simulink model "SRM_ZETA_PID"  (R2020a)
settings: Solver=VariableStepAuto  StartTime=0.0  StopTime=10.0  RelTol=1e-3
undefined symbols (not defined in the file): DiscIntNeverNeededParam, find_system, K, TL, Ts
libraries: powerlib x59
settings Model: Creator=mahfo  LastModifiedBy=mahfo

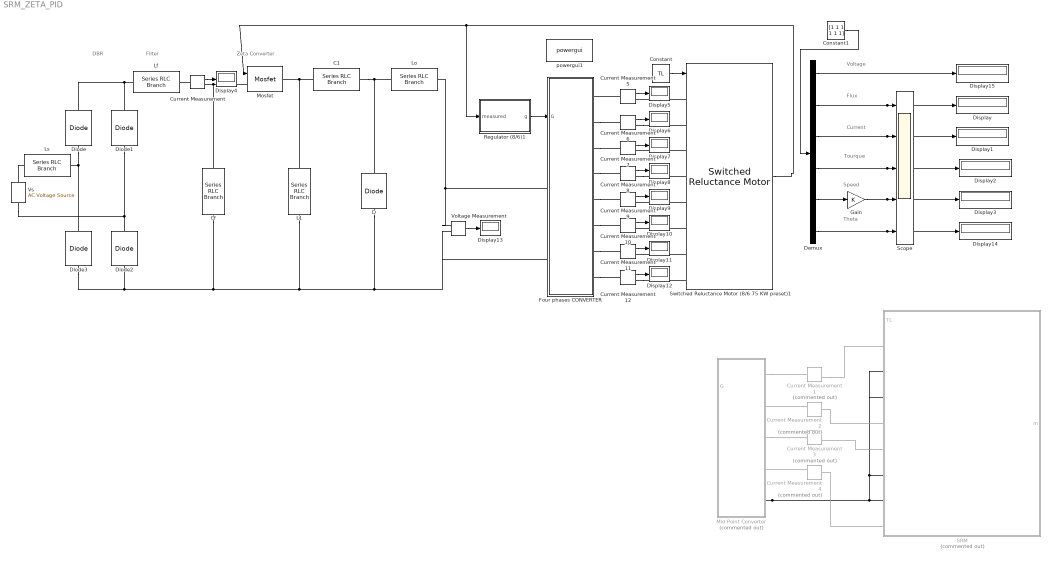
== system SRM_ZETA_PID ==
  note: Flux
  note: DBR
  note: Filter
  note: Zeta Converter
  note: Speed
  note: Theta
  note: Current
  note: Tourque
  note: Voltage
  C1 : powerlib/Elements/Series RLC Branch  LConnTagsString=__new0  RConnTagsString=__new0  BranchType=C  Resistance=1  Inductance=1e-3  SetiL0=off  InitialCurrent=0  Capacitance=1e-6  Setx0=off  InitialVoltage=0  Measurements=None
  Cf : powerlib/Elements/Series RLC Branch  LConnTagsString=__new0  RConnTagsString=__new0  BranchType=C  Resistance=1  Inductance=1e-3  SetiL0=off  InitialCurrent=0  Capacitance=1e-6  Setx0=off  InitialVoltage=0  Measurements=None
  Constant : Constant  Value=TL
  Constant1 : Constant  Value=[1 1 1 1 1 1]
  Current Measurement{,5..12} (9 alike) : powerlib/Measurements/Current Measurement  PhasorSimulation=off  OutputType=Complex  PSBequivalent=0
  Current Measurement{1..4} (4 alike) : powerlib/Measurements/Current Measurement  Commented=on  PhasorSimulation=off  OutputType=Complex  PSBequivalent=0
  D : powerlib/Power Electronics/Diode  Ron=0.001  Lon=0  Vf=0.8  IC=0  UseSnubber=0  Rs=500  Cs=250e-9  Measurements=off
  Demux : Demux  Outputs=6
  Diode{,1..3} (4 alike) : powerlib/Power Electronics/Diode  Ron=0.001  Lon=0  Vf=0.8  IC=0  UseSnubber=0  Rs=500  Cs=250e-9  Measurements=off
  Display{,1..15} (16 alike) : Display
  Four phases CONVERTER : Subsystem  LoadFcn=find_system(gcs,'FollowLinks', 'on', 'LookUnderMasks', 'all');
  Gain : Gain  Gain=K
  L1 : powerlib/Elements/Series RLC Branch  LConnTagsString=__new0  RConnTagsString=__new0  BranchType=L  Resistance=1  Inductance=1e-3  SetiL0=off  InitialCurrent=0  Capacitance=1e-6  Setx0=off  InitialVoltage=0  Measurements=None
  Lf : powerlib/Elements/Series RLC Branch  LConnTagsString=__new0  RConnTagsString=__new0  BranchType=L  Resistance=1  Inductance=1e-3  SetiL0=off  InitialCurrent=0  Capacitance=1e-6  Setx0=off  InitialVoltage=0  Measurements=None
  Lo : powerlib/Elements/Series RLC Branch  LConnTagsString=__new0  RConnTagsString=__new0  BranchType=L  Resistance=1  Inductance=1e-3  SetiL0=off  InitialCurrent=0  Capacitance=1e-6  Setx0=off  InitialVoltage=0  Measurements=None
  Ls : powerlib/Elements/Series RLC Branch  LConnTagsString=__new0  RConnTagsString=__new0  BranchType=L  Resistance=1  Inductance=1e-3  SetiL0=off  InitialCurrent=0  Capacitance=1e-6  Setx0=off  InitialVoltage=0  Measurements=None
  Mid Point Converter : Subsystem  Commented=on
  Mosfet : powerlib/Power Electronics/Mosfet  Ron=0.1  Lon=0  Rd=0.01  Vfd=0  IC=0  Rs=1e5  Cs=inf  Measurements=off
  Regulator (8/6)1 : Subsystem  mask{Iref=50, initpos=[0,-15,-30,-45], TurnOn=37.5, TurnOff=52.5}
      mask prompts: Iref "Reference current"; initpos "initial positions"; TurnOn "Turn-on angle (deg)"; TurnOff "Turn-off angle (deg)"
  SRM : Subsystem  Commented=on
      mask Display: image('F:\Semester 10\Electric Drives\Project\SRM.png'); % Use "Edit Image" on toolstrip to change.
  Scope : Scope  NumInputPorts=5
  Switched Reluctance Motor (8/6 75 KW preset)1 : powerlib/Machines/Switched Reluctance Motor  MachineType="8/6  (75 kw preset model)"  StatorResistance=0.05  Inertia=0.01  Friction=0.005  InitialSpeed=[0,0]  TsPowergui=0  TsBlock=Ts  MachineModel=Specific model  Lq=0.67e-3  Ld=23.6e-3  Lsat=0.15e-3  MaximumCurrent=450  MaximumFluxLinkage=0.486  Source=Dialog  MagnetisationCharacteristic=FTBL  RotorAngleVector=RotorAngles  StatorCurrentVector=StatorCurrents  PlotCurves=off
      settings: SourceProductBaseCode=MT,PS
  Voltage Measurement : powerlib/Measurements/Voltage Measurement  PhasorSimulation=off  OutputType=Complex  PSBequivalent=0
  Vs : powerlib/Electrical Sources/AC Voltage Source  Amplitude=240  Phase=0  Frequency=60  SampleTime=0  Measurements=None  BusType=swing  Pref=10e3  Qref=0  Qmin=-inf  Qmax=+inf
  powergui1 : powerlib/powergui  Priority=1  SimulationMode=Discrete  SampleTime=50e-6  frequency=60  Iterations=50  frequencyindice=60  Pbase=100e6  ErrMax=1e-4  UnitsV=kV  UnitsW=MW  buscounter=0  FunctionMessages=off  echomessages=off  EnableUseOfTLC=off  CurrentSourceSwitches=off  DisableSnubberDevices=off  DisableRonSwitches=off  DisableVfSwitches=off  DisplayEquations=off  AutomaticDiscreteSolvers=off  SolverType=Tustin/Backward Euler (TBE)  Interpol=off  ExternalGateDelay=off  methode=off  Ts=100  x0status=blocks  SPID=on  SwTol=0  HookPort=off  NonlinearTolerance=1e-4  nMaxIteration=100  ContinueOnMaxIteration=off  RestoreLinks=warning  ResistiveCurrentMeasurement=off  Frange=[0:2:500]  Ylog=off  Xlog=on  ShowGrid=off  save=off  variable=ZData  structure=0  ZoomFFT=off  StartTime=0.0  cycles=1  DisplayStyle=1  fundamental=60  FreqAxis=off  MaxFrequency=1000  frequencyindicesteady=1  RmsSteady=1  display=off
  wires:
  Switched Reluctance Motor (8/6 75 KW preset)1/1 -> Regulator (8/6)1/1(measured), Mosfet/1
  Gain/1 -> Display3/1, Scope/4
  Regulator (8/6)1/1(g) -> Four phases CONVERTER/1(G)
  Constant/1 -> Switched Reluctance Motor (8/6 75 KW preset)1/1
  Current Measurement/1 -> Display4/1
  Current Measurement5/1 -> Display5/1
  Current Measurement6/1 -> Display6/1
  Current Measurement7/1 -> Display7/1
  Current Measurement8/1 -> Display8/1
  Current Measurement9/1 -> Display9/1
  Current Measurement10/1 -> Display10/1
  Current Measurement11/1 -> Display11/1
  Current Measurement12/1 -> Display12/1
  Voltage Measurement/1 -> Display13/1
  Demux/6 -> Display14/1, Scope/5
  Demux/5 -> Gain/1
  Demux/4 -> Display2/1, Scope/3
  Demux/3 -> Display1/1, Scope/2
  Demux/2 -> Display/1, Scope/1
  Demux/1 -> Display15/1
  Constant1/1 -> Demux/1
  connections:
  Vs/RConn1 -- Ls/LConn1
  Diode/LConn1 -- Ls/RConn1 -- Diode3/RConn1
  Diode1/LConn1 -- Vs/LConn1 -- Diode2/RConn1
  Diode/RConn1 -- Diode1/RConn1 -- Lf/LConn1
  Diode3/LConn1 -- Cf/RConn1 -- Voltage Measurement/LConn2 -- Four phases CONVERTER/LConn2 -- D/LConn1 -- L1/LConn1 -- Diode2/LConn1
  Current Measurement/LConn1 -- Lf/RConn1
  Current Measurement/RConn1 -- Cf/LConn1 -- Mosfet/LConn1
  L1/RConn1 -- C1/LConn1 -- Mosfet/RConn1
  Lo/LConn1 -- C1/RConn1 -- D/RConn1
  Voltage Measurement/LConn1 -- Lo/RConn1 -- Four phases CONVERTER/LConn1
  Mid Point Converter/RConn5 -- SRM/LConn7 -- SRM/LConn6 -- SRM/LConn3 -- SRM/LConn2
  Current Measurement1/RConn1 -- SRM/LConn1
  Current Measurement2/RConn1 -- Mid Point Converter/RConn2
  SRM/LConn4 -- Current Measurement2/LConn1
  SRM/LConn8 -- Current Measurement4/LConn1
  SRM/LConn5 -- Current Measurement3/RConn1
  Current Measurement4/RConn1 -- Mid Point Converter/RConn4
  Mid Point Converter/RConn3 -- Current Measurement3/LConn1
  Mid Point Converter/RConn1 -- Current Measurement1/LConn1
  Current Measurement5/LConn1 -- Four phases CONVERTER/RConn1
  Switched Reluctance Motor (8/6 75 KW preset)1/LConn1 -- Current Measurement5/RConn1
  Four phases CONVERTER/RConn2 -- Current Measurement6/LConn1
  Current Measurement6/RConn1 -- Switched Reluctance Motor (8/6 75 KW preset)1/LConn2
  Four phases CONVERTER/RConn4 -- Current Measurement8/LConn1
  Switched Reluctance Motor (8/6 75 KW preset)1/LConn3 -- Current Measurement7/RConn1
  Current Measurement8/RConn1 -- Switched Reluctance Motor (8/6 75 KW preset)1/LConn4
  Four phases CONVERTER/RConn3 -- Current Measurement7/LConn1
  Current Measurement12/RConn1 -- Switched Reluctance Motor (8/6 75 KW preset)1/LConn8
  Switched Reluctance Motor (8/6 75 KW preset)1/LConn7 -- Current Measurement11/RConn1
  Four phases CONVERTER/RConn8 -- Current Measurement12/LConn1
  Four phases CONVERTER/RConn6 -- Current Measurement10/LConn1
  Four phases CONVERTER/RConn7 -- Current Measurement11/LConn1
  Switched Reluctance Motor (8/6 75 KW preset)1/LConn5 -- Current Measurement9/RConn1
  Switched Reluctance Motor (8/6 75 KW preset)1/LConn6 -- Current Measurement10/RConn1
  Four phases CONVERTER/RConn5 -- Current Measurement9/LConn1

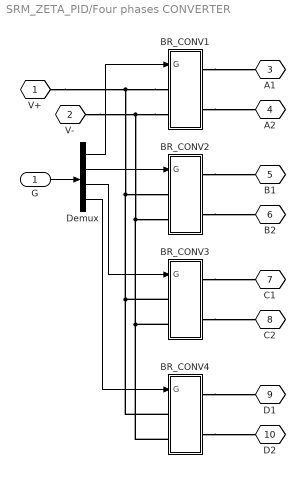
== system SRM_ZETA_PID/Four phases CONVERTER ==
  G : Inport
  BR_CONV1 : Subsystem
  BR_CONV2 : Subsystem
  BR_CONV3 : Subsystem
  BR_CONV4 : Subsystem
  Demux : Demux
      settings: DisplayOption=none
  V+ : PMIOPort  Tag=PMCPort  Side=Left
  V- : PMIOPort  Tag=PMCPort  Port=2  Side=Left
  A1 : PMIOPort  Tag=PMCPort  Port=3  Side=Right
  A2 : PMIOPort  Tag=PMCPort  Port=4  Side=Right
  B1 : PMIOPort  Tag=PMCPort  Port=5  Side=Right
  B2 : PMIOPort  Tag=PMCPort  Port=6  Side=Right
  C1 : PMIOPort  Tag=PMCPort  Port=7  Side=Right
  C2 : PMIOPort  Tag=PMCPort  Port=8  Side=Right
  D1 : PMIOPort  Tag=PMCPort  Port=9  Side=Right
  D2 : PMIOPort  Tag=PMCPort  Port=10  Side=Right
  wires:
  Demux/4 -> BR_CONV4/1(G)
  Demux/3 -> BR_CONV3/1(G)
  Demux/1 -> BR_CONV1/1(G)
  Demux/2 -> BR_CONV2/1(G)
  G/1 -> Demux/1
  connections:
  BR_CONV4/RConn1 -- D1/RConn1
  BR_CONV4/RConn2 -- D2/RConn1
  BR_CONV3/RConn2 -- C2/RConn1
  BR_CONV3/RConn1 -- C1/RConn1
  BR_CONV2/RConn2 -- B2/RConn1
  BR_CONV2/RConn1 -- B1/RConn1
  BR_CONV1/RConn2 -- A2/RConn1
  BR_CONV1/RConn1 -- A1/RConn1
  BR_CONV1/LConn2 -- V-/RConn1 -- BR_CONV3/LConn2 -- BR_CONV4/LConn2 -- BR_CONV2/LConn2
  BR_CONV1/LConn1 -- V+/RConn1 -- BR_CONV3/LConn1 -- BR_CONV4/LConn1 -- BR_CONV2/LConn1

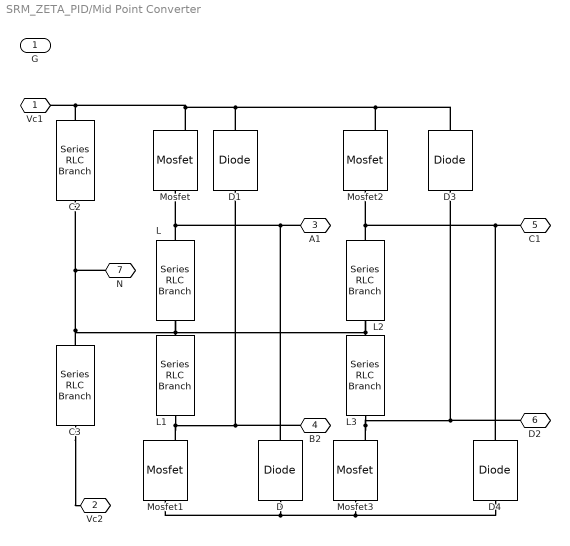
== system SRM_ZETA_PID/Mid Point Converter ==
  G : Inport
  C2 : powerlib/Elements/Series RLC Branch  LConnTagsString=__new0  RConnTagsString=__new0  BranchType=C  Resistance=1  Inductance=1e-3  SetiL0=off  InitialCurrent=0  Capacitance=1e-6  Setx0=off  InitialVoltage=0  Measurements=None
  C3 : powerlib/Elements/Series RLC Branch  LConnTagsString=__new0  RConnTagsString=__new0  BranchType=C  Resistance=1  Inductance=1e-3  SetiL0=off  InitialCurrent=0  Capacitance=1e-6  Setx0=off  InitialVoltage=0  Measurements=None
  D{,1,3..4} (4 alike) : powerlib/Power Electronics/Diode  Ron=0.001  Lon=0  Vf=0.8  IC=0  UseSnubber=0  Rs=500  Cs=250e-9  Measurements=off
  L{,1..3} (4 alike) : powerlib/Elements/Series RLC Branch  LConnTagsString=__new0  RConnTagsString=__new0  BranchType=L  Resistance=1  Inductance=1e-3  SetiL0=off  InitialCurrent=0  Capacitance=1e-6  Setx0=off  InitialVoltage=0  Measurements=None
  Mosfet{,1..3} (4 alike) : powerlib/Power Electronics/Mosfet  Ron=0.1  Lon=0  Rd=0.01  Vfd=0  IC=0  Rs=1e5  Cs=inf  Measurements=off
  Vc1 : PMIOPort  Side=Left
  Vc2 : PMIOPort  Port=2  Side=Left
  A1 : PMIOPort  Port=3  Side=Right
  B2 : PMIOPort  Port=4  Side=Right
  C1 : PMIOPort  Port=5  Side=Right
  D2 : PMIOPort  Port=6  Side=Right
  N : PMIOPort  Port=7  Side=Right
  connections:
  D1/RConn1 -- Vc1/RConn1 -- C2/LConn1 -- Mosfet/LConn1 -- Mosfet2/LConn1 -- D3/RConn1
  C3/RConn1 -- Vc2/RConn1
  A1/RConn1 -- D/RConn1 -- L/LConn1 -- Mosfet/RConn1
  D1/LConn1 -- L1/LConn1 -- Mosfet1/LConn1 -- B2/RConn1
  D4/RConn1 -- C1/RConn1 -- L2/LConn1 -- Mosfet2/RConn1
  D/LConn1 -- Mosfet1/RConn1 -- Mosfet3/RConn1 -- D4/LConn1
  D3/LConn1 -- L3/LConn1 -- Mosfet3/LConn1 -- D2/RConn1
  N/RConn1 -- C2/RConn1 -- C3/LConn1 -- L1/RConn1 -- L3/RConn1 -- L2/RConn1

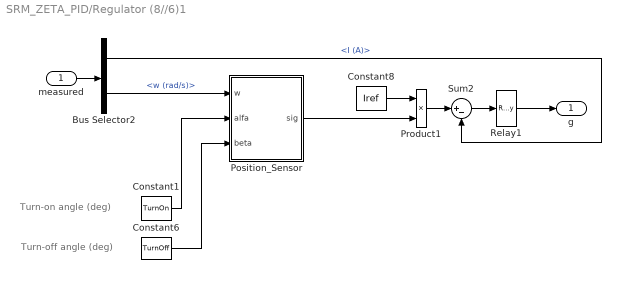
== system SRM_ZETA_PID/Regulator (8//6)1 ==
  note: Turn-on angle (deg)
  note: Turn-off angle (deg)
  measured : Inport
  Bus Selector2 : BusSelector  OutputSignals=I (A),w (rad/s)
  Constant1 : Constant  Value=TurnOn
  Constant6 : Constant  Value=TurnOff
  Constant8 : Constant  Value=Iref
  Position_Sensor : Subsystem
  Product1 : Product  SaturateOnIntegerOverflow=on  OutDataTypeStr=Inherit: Same as first input
  Relay1 : Relay  OnSwitchValue=5  OffSwitchValue=-5  SampleTime=Ts
  Sum2 : Sum  Inputs=|+-  SaturateOnIntegerOverflow=on
  g : Outport  VectorParamsAs1DForOutWhenUnconnected=off
  wires:
  Bus Selector2/2 -> Position_Sensor/1(w)  "<w (rad/s)>"
  Bus Selector2/1 -> Sum2/2  "<I (A)>"
  measured/1 -> Bus Selector2/1
  Relay1/1 -> g/1
  Position_Sensor/1(sig) -> Product1/2
  Constant8/1 -> Product1/1
  Product1/1 -> Sum2/1
  Sum2/1 -> Relay1/1
  Constant6/1 -> Position_Sensor/3(beta)
  Constant1/1 -> Position_Sensor/2(alfa)

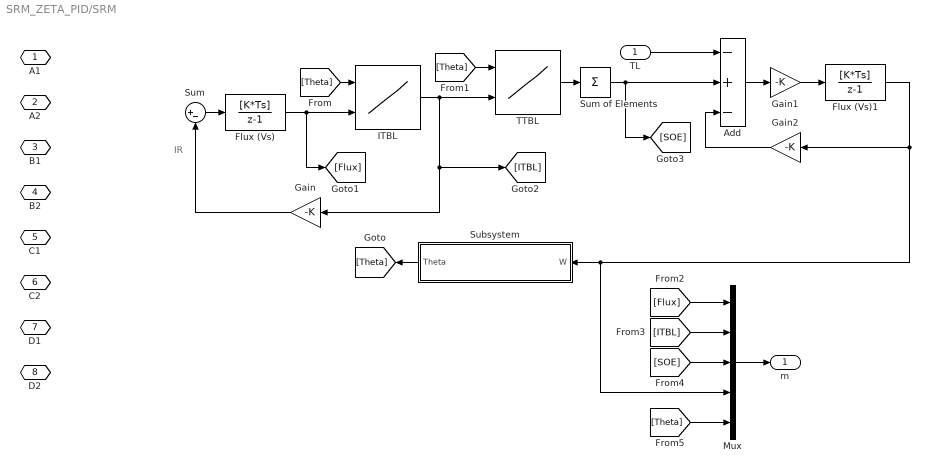
== system SRM_ZETA_PID/SRM ==
  note: IR
  TL : Inport
  Add : Sum  Inputs=-+-
  Flux (Vs) : DiscreteTransferFcn  Numerator=[K*Ts]  Denominator=[1 -1]
  Flux (Vs)1 : DiscreteTransferFcn  Numerator=[K*Ts]  Denominator=[1 -1]
  Gain : Gain  Gain=-K
  Gain1 : Gain  Gain=-K
  Gain2 : Gain  Gain=-K
  ITBL : Lookup_n-D  BreakpointsForDimension1=[1:3]  BreakpointsForDimension2=[1:3]  InternalRulePriority=Speed  RndMeth=Simplest  InputSameDT=on
  Mux : Mux  Inputs=5
  Subsystem : Subsystem
  Sum : Sum  Inputs=|+-
  Sum of Elements : Sum  Inputs=+
  TTBL : Lookup_n-D  BreakpointsForDimension1=[1:3]  BreakpointsForDimension2=[1:3]  InternalRulePriority=Speed  RndMeth=Simplest  InputSameDT=on
  A1 : PMIOPort  Side=Left
  A2 : PMIOPort  Port=2  Side=Left
  B1 : PMIOPort  Port=3  Side=Left
  B2 : PMIOPort  Port=4  Side=Left
  C1 : PMIOPort  Port=5  Side=Left
  C2 : PMIOPort  Port=6  Side=Left
  D1 : PMIOPort  Port=7  Side=Left
  D2 : PMIOPort  Port=8  Side=Left
  m : Outport
  wires:
  Sum/1 -> Flux (Vs)/1
  Flux (Vs)/1 -> [Flux], ITBL/2
  ITBL/1 -> Gain/1, [ITBL], TTBL/2
  TTBL/1 -> Sum of Elements/1
  Gain/1 -> Sum/2
  Sum of Elements/1 -> [SOE], Add/2
  TL/1 -> Add/1
  Add/1 -> Gain1/1
  Gain1/1 -> Flux (Vs)1/1
  Flux (Vs)1/1 -> Mux/4, Subsystem/1(W), Gain2/1
  Gain2/1 -> Add/3
  [Theta] -> ITBL/1
  Subsystem/1(Theta) -> [Theta]
  [Theta] -> TTBL/1
  [Flux] -> Mux/1
  [ITBL] -> Mux/2
  [SOE] -> Mux/3
  [Theta] -> Mux/5
  Mux/1 -> m/1

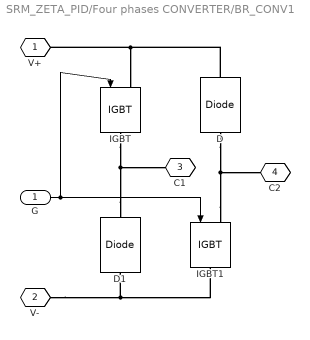
== system SRM_ZETA_PID/Four phases CONVERTER/BR_CONV1 ==
  G : Inport
  D : powerlib/Power Electronics/Diode  Ron=1e-3  Lon=0  Vf=0.8  IC=0  UseSnubber=off  Rs=1000  Cs=inf  Measurements=off
      settings: SourceProductBaseCode=MT,PS
  D1 : powerlib/Power Electronics/Diode  Ron=1e-3  Lon=0  Vf=0.8  IC=0  UseSnubber=off  Rs=1000  Cs=inf  Measurements=off
      settings: SourceProductBaseCode=MT,PS
  IGBT : powerlib/Power Electronics/IGBT  Ron=1e-3  Lon=0  Vf=1  Tf=0  Tt=0  IC=0  Rs=200  Cs=0.1e-6  Measurements=off
      settings: SourceProductBaseCode=MT,PS
  IGBT1 : powerlib/Power Electronics/IGBT  Ron=1e-3  Lon=0  Vf=1  Tf=0  Tt=0  IC=0  Rs=200  Cs=0.1e-6  Measurements=off
      settings: SourceProductBaseCode=MT,PS
  V+ : PMIOPort  Tag=PMCPort  Side=Left
  V- : PMIOPort  Tag=PMCPort  Port=2  Side=Left
  C1 : PMIOPort  Tag=PMCPort  Port=3  Side=Right
  C2 : PMIOPort  Tag=PMCPort  Port=4  Side=Right
  wires:
  G/1 -> IGBT/1, IGBT1/1
  connections:
  D1/LConn1 -- V-/RConn1 -- IGBT1/RConn1
  IGBT1/LConn1 -- D/LConn1 -- C2/RConn1
  D1/RConn1 -- IGBT/RConn1 -- C1/RConn1
  D/RConn1 -- V+/RConn1 -- IGBT/LConn1

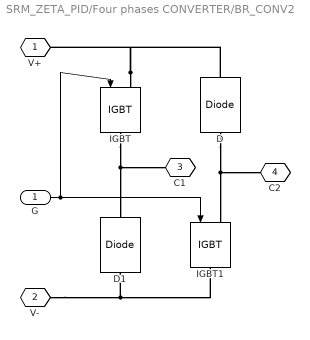
== system SRM_ZETA_PID/Four phases CONVERTER/BR_CONV2 ==
  G : Inport
  D : powerlib/Power Electronics/Diode  Ron=1e-3  Lon=0  Vf=0.8  IC=0  UseSnubber=off  Rs=1000  Cs=inf  Measurements=off
      settings: SourceProductBaseCode=MT,PS
  D1 : powerlib/Power Electronics/Diode  Ron=1e-3  Lon=0  Vf=0.8  IC=0  UseSnubber=off  Rs=1000  Cs=inf  Measurements=off
      settings: SourceProductBaseCode=MT,PS
  IGBT : powerlib/Power Electronics/IGBT  Ron=1e-3  Lon=0  Vf=1  Tf=0  Tt=0  IC=0  Rs=200  Cs=0.1e-6  Measurements=off
      settings: SourceProductBaseCode=MT,PS
  IGBT1 : powerlib/Power Electronics/IGBT  Ron=1e-3  Lon=0  Vf=1  Tf=0  Tt=0  IC=0  Rs=200  Cs=0.1e-6  Measurements=off
      settings: SourceProductBaseCode=MT,PS
  V+ : PMIOPort  Tag=PMCPort  Side=Left
  V- : PMIOPort  Tag=PMCPort  Port=2  Side=Left
  C1 : PMIOPort  Tag=PMCPort  Port=3  Side=Right
  C2 : PMIOPort  Tag=PMCPort  Port=4  Side=Right
  wires:
  G/1 -> IGBT1/1, IGBT/1
  connections:
  IGBT/LConn1 -- V+/RConn1 -- D/RConn1
  IGBT/RConn1 -- D1/RConn1 -- C1/RConn1
  D/LConn1 -- IGBT1/LConn1 -- C2/RConn1
  V-/RConn1 -- D1/LConn1 -- IGBT1/RConn1

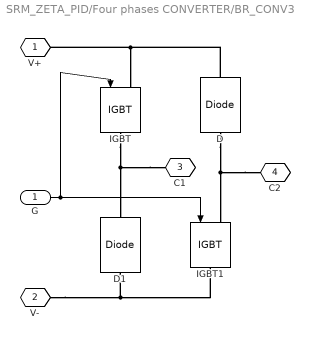
== system SRM_ZETA_PID/Four phases CONVERTER/BR_CONV3 ==
  G : Inport
  D : powerlib/Power Electronics/Diode  Ron=1e-3  Lon=0  Vf=0.8  IC=0  UseSnubber=off  Rs=1000  Cs=inf  Measurements=off
      settings: SourceProductBaseCode=MT,PS
  D1 : powerlib/Power Electronics/Diode  Ron=1e-3  Lon=0  Vf=0.8  IC=0  UseSnubber=off  Rs=1000  Cs=inf  Measurements=off
      settings: SourceProductBaseCode=MT,PS
  IGBT : powerlib/Power Electronics/IGBT  Ron=1e-3  Lon=0  Vf=1  Tf=0  Tt=0  IC=0  Rs=200  Cs=0.1e-6  Measurements=off
      settings: SourceProductBaseCode=MT,PS
  IGBT1 : powerlib/Power Electronics/IGBT  Ron=1e-3  Lon=0  Vf=1  Tf=0  Tt=0  IC=0  Rs=200  Cs=0.1e-6  Measurements=off
      settings: SourceProductBaseCode=MT,PS
  V+ : PMIOPort  Tag=PMCPort  Side=Left
  V- : PMIOPort  Tag=PMCPort  Port=2  Side=Left
  C1 : PMIOPort  Tag=PMCPort  Port=3  Side=Right
  C2 : PMIOPort  Tag=PMCPort  Port=4  Side=Right
  wires:
  G/1 -> IGBT/1, IGBT1/1
  connections:
  IGBT1/RConn1 -- D1/LConn1 -- V-/RConn1
  C2/RConn1 -- IGBT1/LConn1 -- D/LConn1
  C1/RConn1 -- D1/RConn1 -- IGBT/RConn1
  D/RConn1 -- V+/RConn1 -- IGBT/LConn1

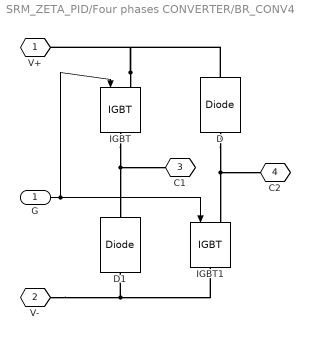
== system SRM_ZETA_PID/Four phases CONVERTER/BR_CONV4 ==
  G : Inport
  D : powerlib/Power Electronics/Diode  Ron=1e-3  Lon=0  Vf=0.8  IC=0  UseSnubber=off  Rs=1000  Cs=inf  Measurements=off
      settings: SourceProductBaseCode=MT,PS
  D1 : powerlib/Power Electronics/Diode  Ron=1e-3  Lon=0  Vf=0.8  IC=0  UseSnubber=off  Rs=1000  Cs=inf  Measurements=off
      settings: SourceProductBaseCode=MT,PS
  IGBT : powerlib/Power Electronics/IGBT  Ron=1e-3  Lon=0  Vf=1  Tf=0  Tt=0  IC=0  Rs=200  Cs=0.1e-6  Measurements=off
      settings: SourceProductBaseCode=MT,PS
  IGBT1 : powerlib/Power Electronics/IGBT  Ron=1e-3  Lon=0  Vf=1  Tf=0  Tt=0  IC=0  Rs=200  Cs=0.1e-6  Measurements=off
      settings: SourceProductBaseCode=MT,PS
  V+ : PMIOPort  Tag=PMCPort  Side=Left
  V- : PMIOPort  Tag=PMCPort  Port=2  Side=Left
  C1 : PMIOPort  Tag=PMCPort  Port=3  Side=Right
  C2 : PMIOPort  Tag=PMCPort  Port=4  Side=Right
  wires:
  G/1 -> IGBT1/1, IGBT/1
  connections:
  IGBT/LConn1 -- V+/RConn1 -- D/RConn1
  IGBT/RConn1 -- D1/RConn1 -- C1/RConn1
  D/LConn1 -- IGBT1/LConn1 -- C2/RConn1
  V-/RConn1 -- D1/LConn1 -- IGBT1/RConn1

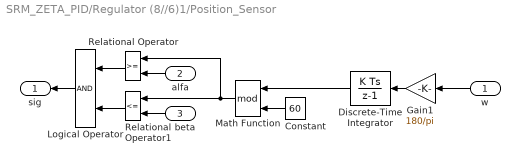
== system SRM_ZETA_PID/Regulator (8//6)1/Position_Sensor ==
  w : Inport
  alfa : Inport  Port=2
  beta : Inport  Port=3
  Constant : Constant  Value=60
  Discrete-Time Integrator : DiscreteIntegrator  InitialCondition=initpos  SampleTime=Ts  ICPrevOutput=DiscIntNeverNeededParam  ICPrevScaledInput=DiscIntNeverNeededParam
  Gain1 : Gain  Gain=180/pi  SaturateOnIntegerOverflow=on  OutDataTypeStr=Inherit: Same as input  ParamDataTypeStr=Inherit: Same as input
  Logical Operator : Logic  AllPortsSameDT=off
  Math Function : Math  Operator=mod  SignedPower=on  SaturateOnIntegerOverflow=on
  Relational Operator : RelationalOperator  RndMeth=Nearest
  Relational Operator1 : RelationalOperator  Operator=<=  RndMeth=Nearest
  sig : Outport  VectorParamsAs1DForOutWhenUnconnected=off
  wires:
  Logical Operator/1 -> sig/1
  w/1 -> Gain1/1
  Math Function/1 -> Relational Operator/1, Relational Operator1/1
  Relational Operator1/1 -> Logical Operator/2
  Gain1/1 -> Discrete-Time Integrator/1
  beta/1 -> Relational Operator1/2
  alfa/1 -> Relational Operator/2
  Relational Operator/1 -> Logical Operator/1
  Constant/1 -> Math Function/2
  Discrete-Time Integrator/1 -> Math Function/1

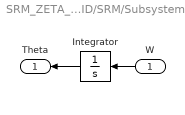
== system SRM_ZETA_PID/SRM/Subsystem ==
  W : Inport
  Integrator : Integrator
  Theta : Outport
  wires:
  Integrator/1 -> Theta/1
  W/1 -> Integrator/1
